simulink model "system_sl"  (R2022b)
settings: Solver=FixedStepAuto  StartTime=0.0  StopTime=tfin  FixedStep=Ts  RelTol=1e-3
values from neighbouring files (symbols this model uses):
  dc = 99    [main.m]
  k = 0.05    [main.m]
  td = 0.015    [main.m]
  Tpwm = 1/w_40    (= 0.0015037593985)    [main.m]
settings Model: Creator=Atti  LastModifiedBy=Atti

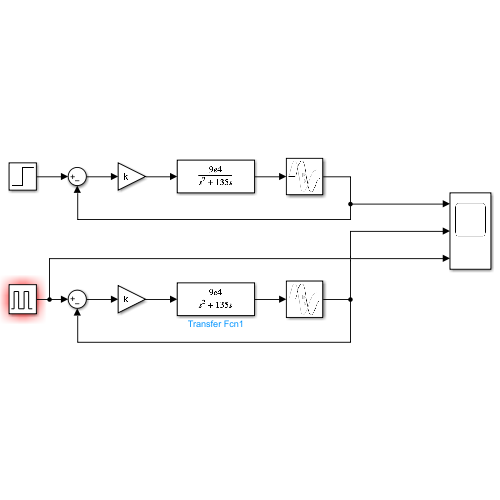
[thumbnail: Simulink's stored preview of the top-level diagram]
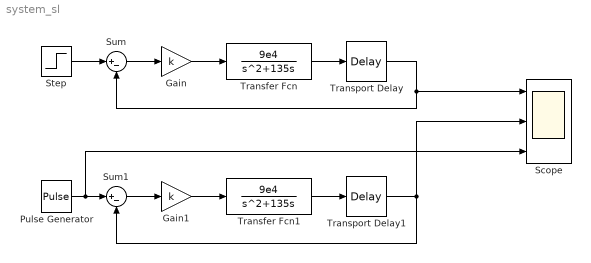
== system system_sl ==
  Gain : Gain  Gain=k
  Gain1 : Gain  Gain=k
  Pulse Generator : DiscretePulseGenerator  PulseType=Time based  Period=Tpwm  PulseWidth=dc
  Scope : Scope  NumInputPorts=3
  Step : Step  Time=0  SampleTime=0
  Sum : Sum  Inputs=|+-
  Sum1 : Sum  Inputs=|+-
  Transfer Fcn : TransferFcn  Numerator=9e4  Denominator=[1 135 0]
  Transfer Fcn1 : TransferFcn  Numerator=9e4  Denominator=[1 135 0]
  Transport Delay : TransportDelay  DelayTime=td
  Transport Delay1 : TransportDelay  DelayTime=td
  wires:
  Step/1 -> Sum/1
  Sum/1 -> Gain/1
  Gain/1 -> Transfer Fcn/1
  Transfer Fcn/1 -> Transport Delay/1
  Transport Delay/1 -> Sum/2, Scope/1
  Transport Delay1/1 -> Scope/2, Sum1/2
  Sum1/1 -> Gain1/1
  Transfer Fcn1/1 -> Transport Delay1/1
  Pulse Generator/1 -> Scope/3, Sum1/1
  Gain1/1 -> Transfer Fcn1/1
